simulink model "dc_machine"  (R2024a)
settings: Solver=VariableStepAuto  StartTime=0.0  StopTime=150  RelTol=1e-3
libraries: simulink x1
settings Model: Creator=emanuele  LastModifiedBy=emanuele

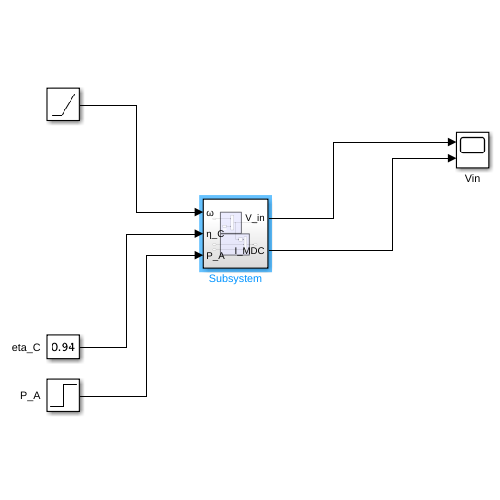
[thumbnail: Simulink's stored preview of the top-level diagram]
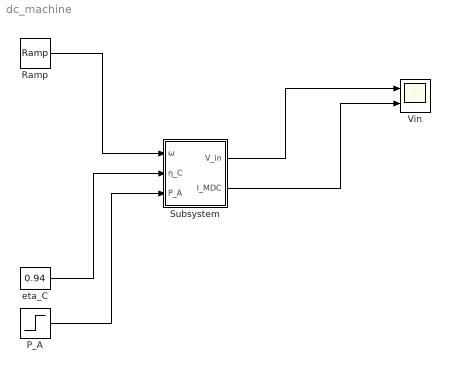
== system dc_machine ==
  P_A : Step  Time=70  After=1000  SampleTime=0
  Ramp : simulink/Sources/Ramp  slope=10  start=10  InitialOutput=0
  Subsystem : Subsystem
  Vin : Scope  NumInputPorts=2
  eta_C : Constant  Value=0.94
  wires:
  Ramp/1 -> Subsystem/1(ω)
  eta_C/1 -> Subsystem/2(η_C)
  P_A/1 -> Subsystem/3(P_A)
  Subsystem/1(V_in) -> Vin/1
  Subsystem/2(I_MDC) -> Vin/2

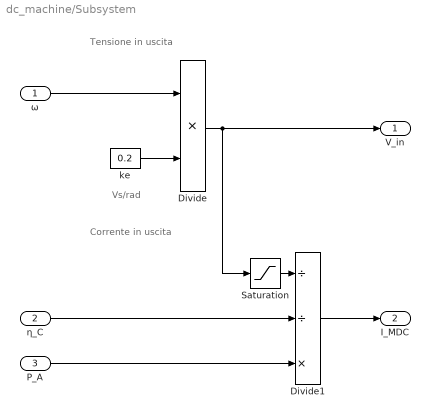
== system dc_machine/Subsystem ==
  note: Corrente in uscita
  note: Vs/rad
  note: Tensione in uscita
  ω : Inport
  η_C : Inport  Port=2
  P_A : Inport  Port=3
  Divide : Product
  Divide1 : Product  Inputs=//*
  Saturation : Saturate  UpperLimit=1000  LowerLimit=1
  ke : Constant  Value=0.2
  V_in : Outport
  I_MDC : Outport  Port=2
  wires:
  ke/1 -> Divide/2
  η_C/1 -> Divide1/2
  Saturation/1 -> Divide1/1
  Divide1/1 -> I_MDC/1
  ω/1 -> Divide/1
  Divide/1 -> V_in/1, Saturation/1
  P_A/1 -> Divide1/3
